simulink model "nonlinear_model_IP"  (R2025b)
settings: Solver=ode4  StartTime=0.0  StopTime=10  FixedStep=1e-3  MaxStep=1e-3  RelTol=1e-3
values from neighbouring files (symbols this model uses):
  b = 0.00007892    (= 7.892e-05)    [IP.m]    (also in Init_Setup_LQRArd.m)
  c = 0.63    [IP.m]    (also in Init_Setup_LQRArd.m)
  g = 9.81    [IP.m]    (also in Init_Setup_LQRArd.m)
  I = (1/12)*(m*(2*l)^2)    (= 0.0009)    [IP.m]    (also in Init_Setup_LQRArd.m)
  Kd = dlqr(Ad,Bd,Q,R)    [IP.m]
  KK = lqr(A,B,Q,R)    [IP.m]    (also in Init_Setup_LQRArd.m)
  l = 0.15    [IP.m]    (also in Init_Setup_LQRArd.m)
  m = 0.12    [IP.m]    (also in Init_Setup_LQRArd.m)
  M_c = 0.5178    [IP.m]    (also in Init_Setup_LQRArd.m = 0.8145)
settings Model: Creator=user  LastModifiedBy=marc-e15
settings DataIOCC: ReturnWorkspaceOutputs=off
settings OptimizationCC: ReuseModelBlockBuffer=off
settings RTWCC: GPUComputeCapability=3.5

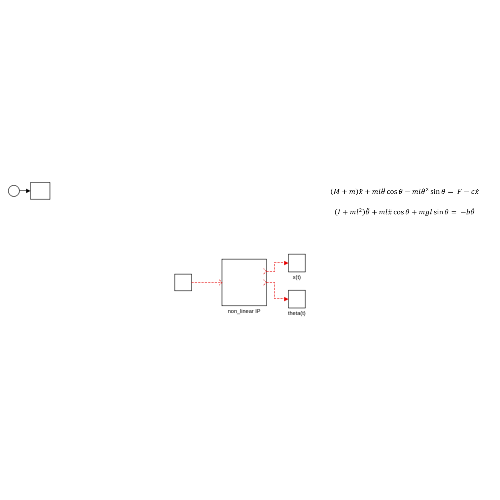
[thumbnail: Simulink's stored preview of the top-level diagram]
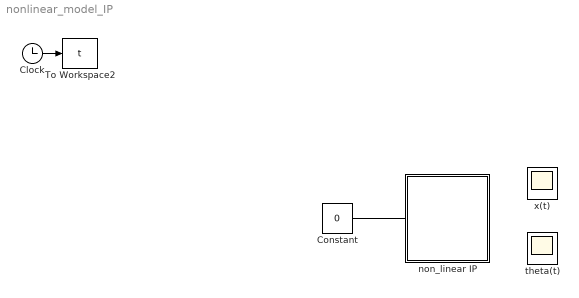
== system nonlinear_model_IP ==
  Clock : Clock
  Constant : Constant  Value=0
  To Workspace2 : ToWorkspace  VariableName=t  SampleTime=-1
  non_linear IP : Subsystem
  theta(t) : Scope
      settings: ActiveDisplayYMinimum=3.0891  ActiveDisplayYMaximum=3.2059
  x(t) : Scope
      settings: ActiveDisplayYMinimum=-0.0948  ActiveDisplayYMaximum=0.09324
  wires:
  Clock/1 -> To Workspace2/1
  ? -> x(t)/1
  ? -> theta(t)/1
  Constant/1 -> ?

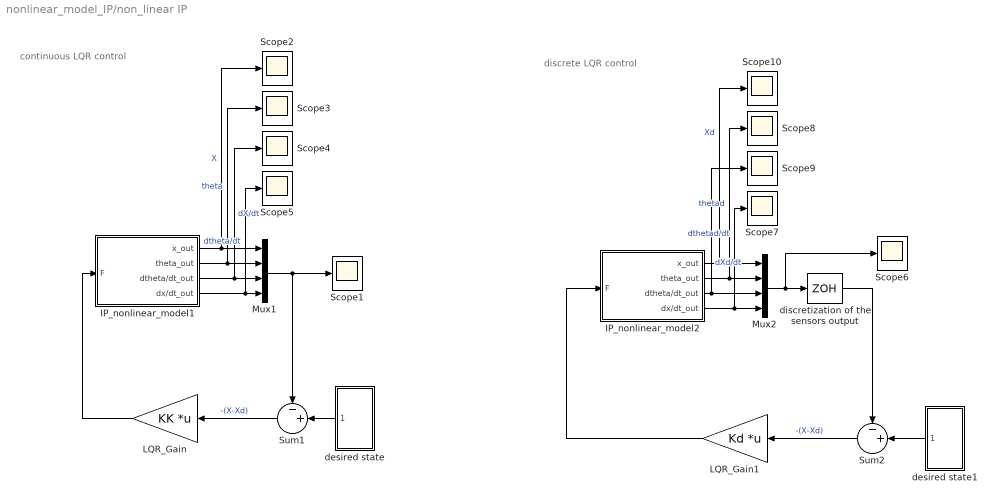
== system nonlinear_model_IP/non_linear IP ==
  note: discrete LQR control
  note: continuous LQR control
  IP_nonlinear_model1 : Subsystem
  IP_nonlinear_model2 : Subsystem
  LQR_Gain : Gain  Gain=KK  Multiplication=Matrix(K*u)
  LQR_Gain1 : Gain  Gain=Kd  Multiplication=Matrix(K*u)
  Mux1 : Mux
  Mux2 : Mux
  Scope{1..10} (10 alike) : Scope
      Scope1 settings: ActiveDisplayYMinimum=-20.63129  ActiveDisplayYMaximum=6.69839
      Scope10 settings: ActiveDisplayYMinimum=-20.63129  ActiveDisplayYMaximum=6.69839  DataLoggingVariableName=ScopeData10
      Scope2 settings: ActiveDisplayYMinimum=-0.1559  ActiveDisplayYMaximum=0.01856  DataLoggingVariableName=ScopeData2
      Scope3 settings: ActiveDisplayYMinimum=2.7742  ActiveDisplayYMaximum=3.57027  DataLoggingVariableName=ScopeData3
      Scope4 settings: ActiveDisplayYMinimum=-4.38534  ActiveDisplayYMaximum=1.37738  DataLoggingVariableName=ScopeData4
      Scope5 settings: ActiveDisplayYMinimum=-20.63129  ActiveDisplayYMaximum=6.69839  DataLoggingVariableName=ScopeData5
      Scope6 settings: ActiveDisplayYMinimum=-20.63129  ActiveDisplayYMaximum=6.69839  DataLoggingVariableName=ScopeData6
      Scope7 settings: ActiveDisplayYMinimum=-20.63129  ActiveDisplayYMaximum=6.69839  DataLoggingVariableName=ScopeData7
      Scope8 settings: ActiveDisplayYMinimum=2.7723  ActiveDisplayYMaximum=3.57048  DataLoggingVariableName=ScopeData8
      Scope9 settings: ActiveDisplayYMinimum=-20.63129  ActiveDisplayYMaximum=6.69839  DataLoggingVariableName=ScopeData9
  Sum1 : Sum  Inputs=-+|
  Sum2 : Sum  Inputs=-+|
  desired state : Subsystem
  desired state1 : Subsystem
  "discretization of the sensors output " : ZeroOrderHold  SampleTime=0.005
  wires:
  IP_nonlinear_model1/1(x_out) -> Scope2/1, Mux1/1  "X"
  IP_nonlinear_model1/2(theta_out) -> Scope3/1, Mux1/2  "theta"
  IP_nonlinear_model1/3(dtheta/dt_out) -> Scope4/1, Mux1/3  "dX/dt"
  IP_nonlinear_model1/4(dx/dt_out) -> Scope5/1, Mux1/4  "dtheta/dt"
  Mux1/1 -> Sum1/1, Scope1/1
  LQR_Gain/1 -> IP_nonlinear_model1/1(F)
  Sum1/1 -> LQR_Gain/1  "-(X-Xd)"
  desired state/1(Out1) -> Sum1/2
  IP_nonlinear_model2/4(dx/dt_out) -> Mux2/4, Scope7/1  "dthetad/dt"
  IP_nonlinear_model2/2(theta_out) -> Scope8/1, Mux2/2  "thetad"
  IP_nonlinear_model2/3(dtheta/dt_out) -> Mux2/3, Scope9/1  "dXd/dt"
  IP_nonlinear_model2/1(x_out) -> Scope10/1, Mux2/1  "Xd"
  Mux2/1 -> Scope6/1, "discretization of the sensors output "/1
  "discretization of the sensors output "/1 -> Sum2/1
  desired state1/1(Out1) -> Sum2/2
  Sum2/1 -> LQR_Gain1/1  "-(X-Xd)"
  LQR_Gain1/1 -> IP_nonlinear_model2/1(F)

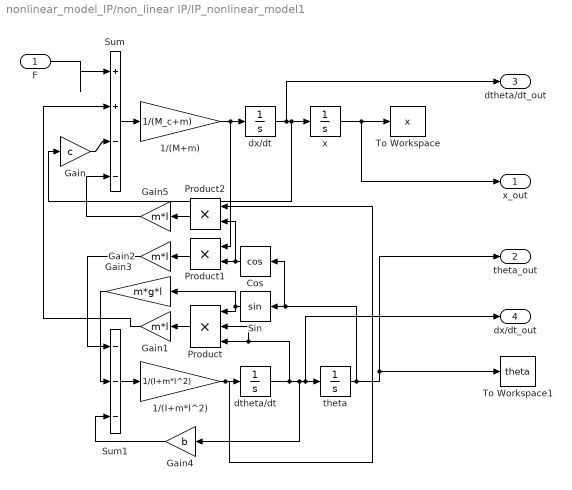
== system nonlinear_model_IP/non_linear IP/IP_nonlinear_model1 ==
  F : Inport
  1/(I+m*l^2) : Gain  Gain=1/(I+m*l^2)
  1/(M+m) : Gain  Gain=1/(M_c+m)
  Cos : Trigonometry  Operator=cos
  Gain : Gain  Gain=c
  Gain1 : Gain  Gain=m*l
  Gain2 : Gain  Gain=m*l
  Gain3 : Gain  Gain=m*g*l
  Gain4 : Gain  Gain=b
  Gain5 : Gain  Gain=m*l
  Product : Product  Inputs=3
  Product1 : Product
  Product2 : Product
  Sin : Trigonometry
  Sum : Sum  Inputs=|++--
  Sum1 : Sum  Inputs=---
  To Workspace : ToWorkspace  VariableName=x  SaveFormat=Structure With Time  SampleTime=-1
  To Workspace1 : ToWorkspace  VariableName=theta  SaveFormat=Structure With Time  SampleTime=-1
  dtheta/dt : Integrator
  dx/dt : Integrator
  theta : Integrator  InitialCondition=pi+20*pi/180
  x : Integrator
  x_out : Outport
  theta_out : Outport  Port=2
  dtheta/dt_out : Outport  Port=3
  dx/dt_out : Outport  Port=4
  wires:
  x/1 -> To Workspace/1, x_out/1
  Product2/1 -> Gain5/1
  Gain/1 -> Sum/3
  Gain1/1 -> Sum/2
  Gain3/1 -> Sum1/2
  F/1 -> Sum/1
  theta/1 -> Sin/1, Cos/1, To Workspace1/1, theta_out/1
  Sum1/1 -> 1/(I+m*l^2)/1
  Product/1 -> Gain1/1
  Gain2/1 -> Sum1/1
  1/(I+m*l^2)/1 -> dtheta/dt/1, Product2/1
  Product1/1 -> Gain2/1
  Gain5/1 -> Sum/4
  dx/dt/1 -> x/1, Gain/1, dtheta/dt_out/1
  Sin/1 -> Product/1, Gain3/1
  Sum/1 -> 1/(M+m)/1
  dtheta/dt/1 -> theta/1, dx/dt_out/1, Gain4/1, Product/3, Product/2
  Gain4/1 -> Sum1/3
  Cos/1 -> Product1/2, Product2/2
  1/(M+m)/1 -> dx/dt/1, Product1/1

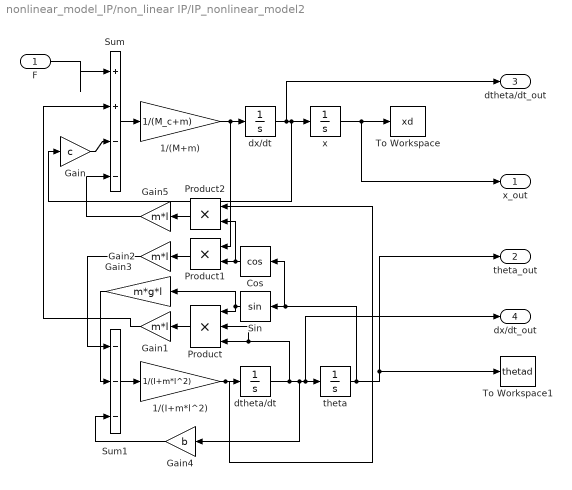
== system nonlinear_model_IP/non_linear IP/IP_nonlinear_model2 ==
  F : Inport
  1/(I+m*l^2) : Gain  Gain=1/(I+m*l^2)
  1/(M+m) : Gain  Gain=1/(M_c+m)
  Cos : Trigonometry  Operator=cos
  Gain : Gain  Gain=c
  Gain1 : Gain  Gain=m*l
  Gain2 : Gain  Gain=m*l
  Gain3 : Gain  Gain=m*g*l
  Gain4 : Gain  Gain=b
  Gain5 : Gain  Gain=m*l
  Product : Product  Inputs=3
  Product1 : Product
  Product2 : Product
  Sin : Trigonometry
  Sum : Sum  Inputs=|++--
  Sum1 : Sum  Inputs=---
  To Workspace : ToWorkspace  VariableName=xd  SaveFormat=Structure With Time  SampleTime=-1
  To Workspace1 : ToWorkspace  VariableName=thetad  SaveFormat=Structure With Time  SampleTime=-1
  dtheta/dt : Integrator
  dx/dt : Integrator
  theta : Integrator  InitialCondition=pi+20*pi/180
  x : Integrator
  x_out : Outport
  theta_out : Outport  Port=2
  dtheta/dt_out : Outport  Port=3
  dx/dt_out : Outport  Port=4
  wires:
  x/1 -> To Workspace/1, x_out/1
  Product2/1 -> Gain5/1
  Gain/1 -> Sum/3
  Gain1/1 -> Sum/2
  Gain3/1 -> Sum1/2
  F/1 -> Sum/1
  theta/1 -> Sin/1, Cos/1, To Workspace1/1, theta_out/1
  Sum1/1 -> 1/(I+m*l^2)/1
  Product/1 -> Gain1/1
  Gain2/1 -> Sum1/1
  1/(I+m*l^2)/1 -> dtheta/dt/1, Product2/1
  Product1/1 -> Gain2/1
  Gain5/1 -> Sum/4
  dx/dt/1 -> x/1, Gain/1, dtheta/dt_out/1
  Sin/1 -> Product/1, Gain3/1
  Sum/1 -> 1/(M+m)/1
  dtheta/dt/1 -> theta/1, dx/dt_out/1, Gain4/1, Product/3, Product/2
  Gain4/1 -> Sum1/3
  Cos/1 -> Product1/2, Product2/2
  1/(M+m)/1 -> dx/dt/1, Product1/1

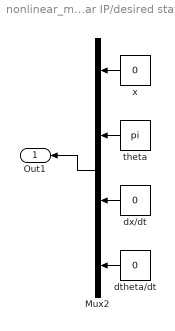
== system nonlinear_model_IP/non_linear IP/desired state ==
  Mux2 : Mux
  dtheta/dt : Constant  Value=0
  dx/dt : Constant  Value=0
  theta : Constant  Value=pi
  x : Constant  Value=0
  Out1 : Outport
  wires:
  dx/dt/1 -> Mux2/3
  theta/1 -> Mux2/2
  Mux2/1 -> Out1/1
  x/1 -> Mux2/1
  dtheta/dt/1 -> Mux2/4

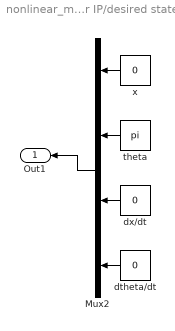
== system nonlinear_model_IP/non_linear IP/desired state1 ==
  Mux2 : Mux
  dtheta/dt : Constant  Value=0
  dx/dt : Constant  Value=0
  theta : Constant  Value=pi
  x : Constant  Value=0
  Out1 : Outport
  wires:
  dx/dt/1 -> Mux2/3
  theta/1 -> Mux2/2
  Mux2/1 -> Out1/1
  x/1 -> Mux2/1
  dtheta/dt/1 -> Mux2/4
